simulink model "buck_duty_limit_anti_windup_logic"  (R2024b)
settings: Solver=ode4  StartTime=0.0  StopTime=0.014  FixedStep=5e-7  RelTol=1e-3
undefined symbols (not defined in the file): DiscIntNeverNeededParam
settings Model: Creator=ww  LastModifiedBy=ww

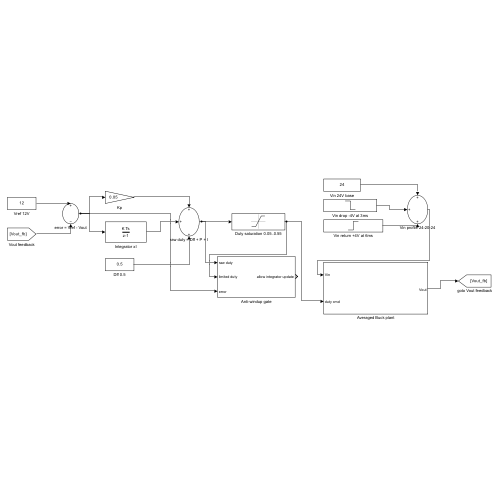
[thumbnail: Simulink's stored preview of the top-level diagram]
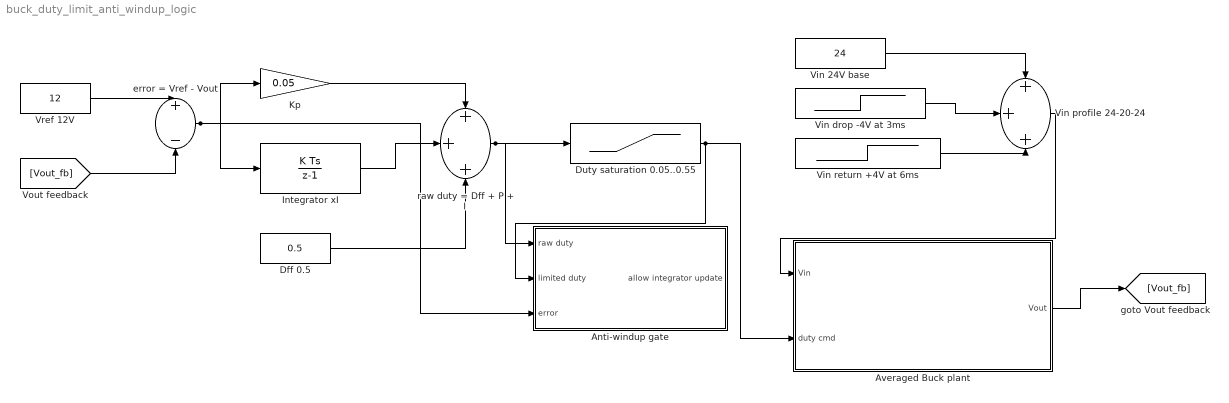
== system buck_duty_limit_anti_windup_logic ==
  Anti-windup gate : Subsystem
  Averaged Buck plant : Subsystem
  Dff 0.5 : Constant  Value=0.5
  Duty saturation 0.05..0.55 : Saturate  UpperLimit=0.55  LowerLimit=0.05
  Integrator xI : DiscreteIntegrator  gainval=200  InitialCondition=0.0041667  SampleTime=5e-6  ICPrevOutput=DiscIntNeverNeededParam  ICPrevScaledInput=DiscIntNeverNeededParam
  Kp : Gain  Gain=0.05
  Vin 24V base : Constant  Value=24
  Vin drop -4V at 3ms : Step  Time=0.003  After=-4  SampleTime=0
  Vin profile 24-20-24 : Sum  Inputs=+++
  Vin return +4V at 6ms : Step  Time=0.006  After=4  SampleTime=0
  Vref 12V : Constant  Value=12
  error = Vref - Vout : Sum  Inputs=+-
  raw duty = Dff + P + I : Sum  Inputs=+++
  wires:
  Vref 12V/1 -> error = Vref - Vout/1
  [Vout_fb] -> error = Vref - Vout/2
  error = Vref - Vout/1 -> Kp/1, Integrator xI/1, Anti-windup gate/3(error)
  Kp/1 -> raw duty = Dff + P + I/1
  Integrator xI/1 -> raw duty = Dff + P + I/2
  Dff 0.5/1 -> raw duty = Dff + P + I/3
  raw duty = Dff + P + I/1 -> Duty saturation 0.05..0.55/1, Anti-windup gate/1(raw duty)
  Duty saturation 0.05..0.55/1 -> Anti-windup gate/2(limited duty), Averaged Buck plant/2(duty cmd)
  Vin 24V base/1 -> Vin profile 24-20-24/1
  Vin drop -4V at 3ms/1 -> Vin profile 24-20-24/2
  Vin return +4V at 6ms/1 -> Vin profile 24-20-24/3
  Vin profile 24-20-24/1 -> Averaged Buck plant/1(Vin)
  Averaged Buck plant/1(Vout) -> [Vout_fb]

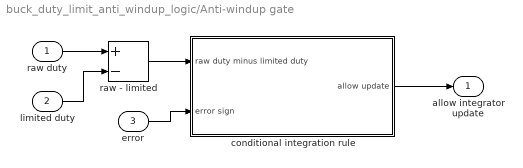
== system buck_duty_limit_anti_windup_logic/Anti-windup gate ==
  raw duty : Inport
  limited duty : Inport  Port=2
  error : Inport  Port=3
  conditional integration rule : Subsystem
  raw - limited : Sum  Inputs=+-
  allow integrator update : Outport
  wires:
  error/1 -> conditional integration rule/2(error sign)
  raw - limited/1 -> conditional integration rule/1(raw duty minus limited duty)
  limited duty/1 -> raw - limited/2
  raw duty/1 -> raw - limited/1
  conditional integration rule/1(allow update) -> allow integrator update/1

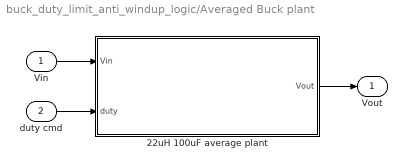
== system buck_duty_limit_anti_windup_logic/Averaged Buck plant ==
  Vin : Inport
  duty cmd : Inport  Port=2
  22uH 100uF average plant : Subsystem
  Vout : Outport
  wires:
  22uH 100uF average plant/1(Vout) -> Vout/1
  duty cmd/1 -> 22uH 100uF average plant/2(duty)
  Vin/1 -> 22uH 100uF average plant/1(Vin)

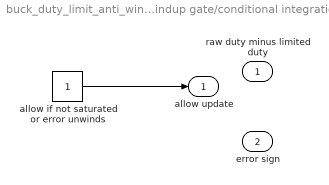
== system buck_duty_limit_anti_windup_logic/Anti-windup gate/conditional integration rule ==
  raw duty minus limited duty : Inport
  error sign : Inport  Port=2
  allow if not saturated or error unwinds : Constant
  allow update : Outport
  wires:
  allow if not saturated or error unwinds/1 -> allow update/1

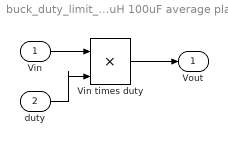
== system buck_duty_limit_anti_windup_logic/Averaged Buck plant/22uH 100uF average plant ==
  Vin : Inport
  duty : Inport  Port=2
  Vin times duty : Product
  Vout : Outport
  wires:
  Vin/1 -> Vin times duty/1
  Vin times duty/1 -> Vout/1
  duty/1 -> Vin times duty/2
